simulink model "Validacion_Motor"  (R2020b)
settings: Solver=FixedStepAuto  StartTime=0.0  StopTime=4  FixedStep=0.02  RelTol=1e-3
libraries: simulink x1
settings Model: Creator=DellXPS13  LastModifiedBy=alexa
settings DataIOCC: ReturnWorkspaceOutputs=off
settings DebuggingCC: ArithmeticOperatorsInVariantConditions=warning
settings SFSimCC: CustomCodeUndefinedFunction=UseInterfaceOnly

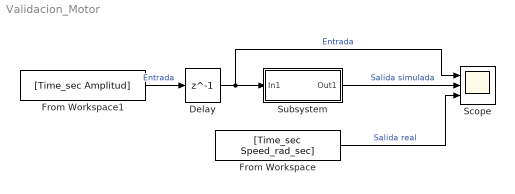
== system Validacion_Motor ==
  Delay : Delay  DelayLength=1
  From Workspace : FromWorkspace  VariableName=[Time_sec Speed_rad_sec]
  From Workspace1 : FromWorkspace  VariableName=[Time_sec Amplitud]
  Scope : Scope  NumInputPorts=3
  Subsystem : Subsystem  mask{k=0.146, tau=0.0634}
      mask prompts: k "K (Voltaje medio x k ajuste curva)"; tau "Constante de tiempo (tau)"
      mask Display: image('icon_tf.png');
  wires:
  Delay/1 -> Scope/1, Subsystem/1(In1)  "Entrada"
  From Workspace/1 -> Scope/3  "Salida real"
  Subsystem/1(Out1) -> Scope/2  "Salida simulada"
  From Workspace1/1 -> Delay/1  "Entrada"

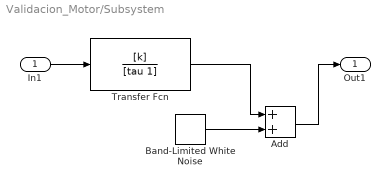
== system Validacion_Motor/Subsystem ==
  In1 : Inport
  Add : Sum
  Band-Limited White Noise : simulink/Sources/Band-Limited White Noise  Cov=[0.002]  Ts=0.02  seed=[23341]
  Transfer Fcn : TransferFcn  Numerator=[k]  Denominator=[tau 1]
  Out1 : Outport  VectorParamsAs1DForOutWhenUnconnected=off
  wires:
  In1/1 -> Transfer Fcn/1
  Transfer Fcn/1 -> Add/1
  Band-Limited White Noise/1 -> Add/2
  Add/1 -> Out1/1
